simulink model "NetworkModelIntermediateIntersectionRDDSample1"  (R2018b)
settings: Solver=VariableStepAuto  StartTime=0.0  StopTime=10.0  RelTol=1e-3
values from neighbouring files (symbols this model uses):
  Ax = [0 1  0   0 ... (first row only)    [DroneSubsystemModelling.m]
  Ay = [0 1  0   0 ... (first row only)    [DroneSubsystemModelling.m]
  Bx = [0;0;0;b1]    [DroneSubsystemModelling.m]
  By = [0;0;0;b2]    [DroneSubsystemModelling.m]
  ConflictDrone1andDrone2 = ControlDetectionFunction(tout,PositionXDrone1TEST, PositionYDrone1TEST, PositionXDrone2TEST, PositionYDrone2TEST, ConflictDrone1andDrone2)    [ConflictDetectionTEST.m]
  ConflictDrone1andDrone3 = ControlDetectionFunction(tout,PositionXDrone1TEST, PositionYDrone1TEST, PositionXDrone3TEST, PositionYDrone3TEST, ConflictDrone1andDrone3)    [ConflictDetectionTEST.m]
  ConflictDrone1andDrone4 = ControlDetectionFunction(tout,PositionXDrone1TEST, PositionYDrone1TEST, PositionXDrone4TEST, PositionYDrone4TEST, ConflictDrone1andDrone4)    [ConflictDetectionTEST.m]
  ConflictDrone2andDrone3 = ControlDetectionFunction(tout,PositionXDrone2TEST, PositionYDrone2TEST, PositionXDrone3TEST, PositionYDrone3TEST, ConflictDrone2andDrone3)    [ConflictDetectionTEST.m]
  ConflictDrone2andDrone4 = ControlDetectionFunction(tout,PositionXDrone2, PositionYDrone2, PositionXDrone4, PositionYDrone4, ConflictDrone2andDrone4)    [ConflictDetection.m]    (also in ConflictDetectionTEST.m = ControlDetectionFunction(tout,PositionXDrone2TEST, PositionY)
  ConflictDrone3andDrone4 = ControlDetectionFunction(tout,PositionXDrone3TEST, PositionYDrone3TEST, PositionXDrone4TEST, PositionYDrone4TEST, ConflictDrone3andDrone4)    [ConflictDetectionTEST.m]
  Cpx = [1 0 0 0]    [DroneSubsystemModelling.m]
  Cpy = [1 0 0 0]    [DroneSubsystemModelling.m]
  Cvx = [0 1 0 0]    [DroneSubsystemModelling.m]
  Cvy = [0 1 0 0]    [DroneSubsystemModelling.m]
  K1 = 1    [MotionModelling.m]
  K2 = 0.25    [MotionModelling.m]
  K3 = 0.25    [MotionModelling.m]
  K4 = 1    [MotionModelling.m]
  theta1 = -180    [MotionModelling.m]
  theta2 = -3*180/4    (= -135)    [MotionModelling.m]
  theta3 = -2*180/4    (= -90)    [MotionModelling.m]
  theta4 = -180/4    (= -45)    [MotionModelling.m]
  VelocityStarX1 = vx10    [MotionModelling.m]
  VelocityStarX2 = vx20    [MotionModelling.m]
  VelocityStarX3 = vx30    [MotionModelling.m]
  VelocityStarX4 = vx40    [MotionModelling.m]
  VelocityStarY1 = vy10    [MotionModelling.m]
  VelocityStarY2 = vy20    [MotionModelling.m]
  VelocityStarY3 = vy30    [MotionModelling.m]
  VelocityStarY4 = vy40    [MotionModelling.m]
  X10 = [x10 vx10 0 0]'    [MotionModelling.m]
  X20 = [x20 vx20 0 0]'    [MotionModelling.m]
  X30 = [x30 vx30 0 0]'    [MotionModelling.m]
  X40 = [x40 vx40 0 0]'    [MotionModelling.m]
  Y10 = [y10 vy10 0 0]'    [MotionModelling.m]
  Y20 = [y20 vy20 0 0]'    [MotionModelling.m]
  Y30 = [y30 vy30 0 0]'    [MotionModelling.m]
  Y40 = [y40 vy40 0 0]'    [MotionModelling.m]
libraries: simulink x8
settings Model: Creator=CowUser  LastModifiedBy=CowUser

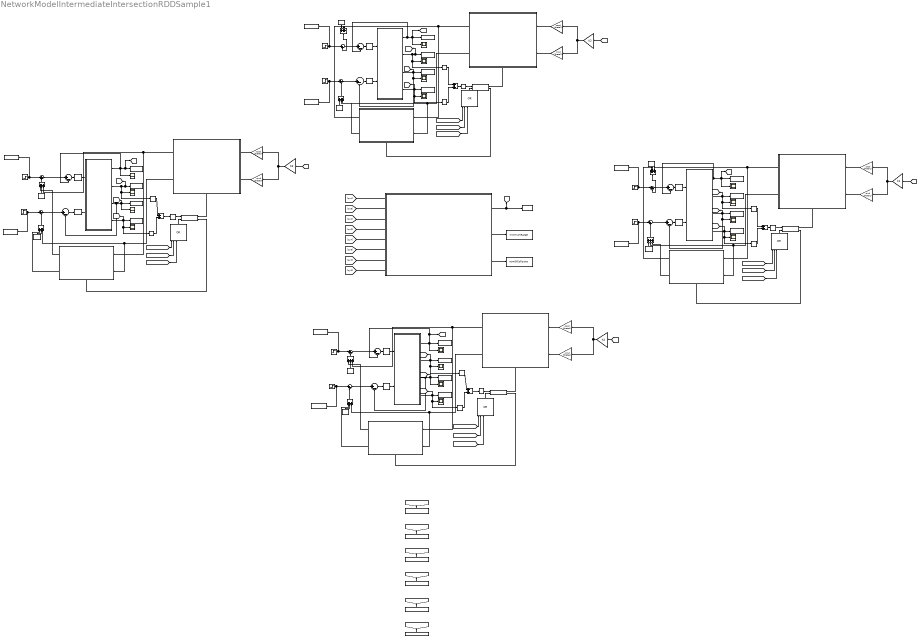
== system NetworkModelIntermediateIntersectionRDDSample1 ==
  note: Drone 3
  note: Drone 1
  note: Drone 2
  note: Drone 4
  note: Sample 4
  note: Sample 2
  note: Sample 1
  note: Sample 3
  note: Sample 5
  note: Sample 6
  Add{7,10..16} (8 alike) : Sum  Inputs=+++
  Add{8..9,17..18} (4 alike) : Sum
  Constant{6..8,10..14} (8 alike) : Constant  Value=0
  Constant25 : Constant  Value=ConflictDrone1andDrone3
  Constant26 : Constant  Value=ConflictDrone1andDrone2
  Constant27 : Constant  Value=ConflictDrone1andDrone4
  Constant28 : Constant  Value=ConflictDrone2andDrone4
  Constant29 : Constant  Value=ConflictDrone3andDrone4
  Constant30 : Constant  Value=ConflictDrone2andDrone3  VectorParams1D=off
  Drone1 Subsystem : Subsystem
  Drone2 Subsystem : Subsystem
  Drone3 Subsystem : Subsystem
  Drone4 Subsystem : Subsystem
  Gain : Gain  Gain=K2
  Gain1 : Gain  Gain=-sind (theta4)
  Gain10 : Gain  Gain=cosd (theta1)
  Gain11 : Gain  Gain=-cosd (theta3)
  Gain12 : Gain  Gain=sind (theta1)
  Gain2 : Gain  Gain=cosd (theta2)
  Gain3 : Gain  Gain=-cosd (theta4)
  Gain4 : Gain  Gain=sind (theta2)
  Gain5 : Gain  Gain=K4
  Gain6 : Gain  Gain=K3
  Gain7 : Gain  Gain=K1
  Gain9 : Gain  Gain=-sind (theta3)
  If Action Subsystem2 : Subsystem  TreatAsAtomicUnit=on
  If Action Subsystem3 : Subsystem  TreatAsAtomicUnit=on
  If Action Subsystem5 : Subsystem  TreatAsAtomicUnit=on
  If Action Subsystem6 : Subsystem  TreatAsAtomicUnit=on
  If{2,4..6} (4 alike) : If  NumInputs=2  IfExpression=(u1 <= R)&(u2 == 1)  ElseIfExpressions=(u1 > R)&(u2 == 1)  ShowElse=off
  MATLAB Function2 : MATLAB Function  TreatAsAtomicUnit=on
  OR{3..6} (4 alike) : Logic  Operator=OR  Inputs=7  IconShape=distinctive  AllPortsSameDT=off  OutDataTypeStr='double'
  PID Controller{2,4..5,8..12} (8 alike) : simulink/Continuous/PID Controller  Controller=PID  Form=Parallel  TimeDomain=Continuous-time  SampleTime=-1  IntegratorMethod=Forward Euler  FilterMethod=Forward Euler  ControllerParametersSource=internal  P=1.97139727738968e-05  I=1.5233344900537e-08  D=0.00566857635684116  UseFilter=on  N=15.1370363747334  TunerSelectOption=Transfer Function Based (PID Tuner App)  InitialConditionSource=internal  InitialConditionForIntegrator=0  InitialConditionForFilter=0  DifferentiatorICPrevScaledInput=0  ExternalReset=none  TrackingMode=off  Kt=1  LimitOutput=off  UpperSaturationLimit=inf  LowerSaturationLimit=-inf  LinearizeAsGain=on  AntiWindupMode=none  Kb=1  POutMin=[]  POutMax=[]  IOutMin=[]  IOutMax=[]  DOutMin=[]  DOutMax=[]  NOutMin=[]  NOutMax=[]  SumOutMin=[]  SumOutMax=[]  SaturationOutMin=[]  SaturationOutMax=[]  PParamMin=[]  PParamMax=[]  IParamMin=[]  IParamMax=[]  DParamMin=[]  DParamMax=[]  NParamMin=[]  NParamMax=[]  KbParamMin=[]  KbParamMax=[]  KtParamMin=[]  KtParamMax=[]  KbOutMin=[]  KbOutMax=[]  KtOutMin=[]  KtOutMax=[]  IntegratorOutMin=[]  IntegratorOutMax=[]  FilterOutMin=[]  FilterOutMax=[]  SumI1OutMin=[]  SumI1OutMax=[]  SumI2OutMin=[]  SumI2OutMax=[]  SumI3OutMin=[]  SumI3OutMax=[]  SumI4OutMin=[]  SumI4OutMax=[]  SumDOutMin=[]  SumDOutMax=[]  DifferentiatorOutMin=[]  DifferentiatorOutMax=[]  FilterDiffOutCoefMin=[]  FilterDiffOutCoefMax=[]  ReciprocalOutMin=[]  ReciprocalOutMax=[]  SumDenOutMin=[]  SumDenOutMax=[]  SumNumOutMin=[]  SumNumOutMax=[]  DivideOutMin=[]  DivideOutMax=[]  IntegratorContinuousStateAttributes=''  IntegratorStateMustResolveToSignalObject=off  IntegratorRTWStateStorageClass=Auto  FilterContinuousStateAttributes=''  FilterStateMustResolveToSignalObject=off  FilterRTWStateStorageClass=Auto  ParallelPVariant=InternalParameters  IdealPVariant=Disabled  IVariant=InternalParameters  DVariant=InternalParameters  IntegratorVariant=Continuous  SatVariant=Disabled  AWVariant=Passthrough  PCopyVariant=Disabled  TRVariant=Disabled  FdbkBlocksVariant=Forward  IdealPFdbkVariant=Disabled  SatFdbkVariant=Disabled  DerivativeFilterVariant=ContFilter  NVariant=InternalParameters  NCopyVariant=Disabled  FilterICVariant=InternalICsFilter  IntegratorICVariant=InternalICs  ExternalResetVariant=Disabled  TRSumVariant=Passthrough  SumFdbkVariant=Disabled  SumVariant=Sum_PID
  PositionXDrone{1..4} (4 alike) : Scope
  PositionYDrone{1..4} (4 alike) : Scope
  Sqrt{3..6} (4 alike) : Sqrt  SaturateOnIntegerOverflow=on
  Square{5..12} (8 alike) : Math  Operator=square  SaturateOnIntegerOverflow=on
  Step 10 : Step  Time=0  After=VelocityStarY1  SampleTime=0
  Step 11 : Step  Time=0  After=VelocityStarX3  SampleTime=0
  Step 12 : Step  Time=0  After=VelocityStarY3  SampleTime=0
  Step 3 : Step  Time=0  After=VelocityStarX2  SampleTime=0
  Step 4 : Step  Time=0  After=VelocityStarY2  SampleTime=0
  Step 5 : Step  Time=0  After=VelocityStarX4  SampleTime=0
  Step 6 : Step  Time=0  After=VelocityStarY4  SampleTime=0
  Step 9 : Step  Time=0  After=VelocityStarX1  SampleTime=0
  Sum{9..24} (16 alike) : Sum  Inputs=|+-
  Switch Case Action Subsystem : Subsystem  TreatAsAtomicUnit=on
  Switch Case Action Subsystem1 : Subsystem  TreatAsAtomicUnit=on
  Switch Case Action Subsystem4 : Subsystem  TreatAsAtomicUnit=on
  Switch Case Action Subsystem5 : Subsystem  TreatAsAtomicUnit=on
  To Workspace10 : ToWorkspace  VariableName=VelocityYDrone4  SampleTime=-1
  To Workspace11 : ToWorkspace  VariableName=PositionXDrone4  SampleTime=-1
  To Workspace12 : ToWorkspace  VariableName=VelocityXDrone4  SampleTime=-1
  To Workspace13 : ToWorkspace  VariableName=VelocityStarX4  SampleTime=-1
  To Workspace14 : ToWorkspace  VariableName=PositionYDrone4  SampleTime=-1
  To Workspace15 : ToWorkspace  VariableName=PositionXDrone2  SampleTime=-1
  To Workspace16 : ToWorkspace  VariableName=VelocityXDrone2  SampleTime=-1
  To Workspace17 : ToWorkspace  VariableName=VelocityStarX2  SampleTime=-1
  To Workspace18 : ToWorkspace  VariableName=PositionYDrone2  SampleTime=-1
  To Workspace25 : ToWorkspace  VariableName=VelocityYDrone3  SampleTime=-1
  To Workspace26 : ToWorkspace  VariableName=VelocityXDrone1  SampleTime=-1
  To Workspace27 : ToWorkspace  VariableName=PositionXDrone3  SampleTime=-1
  To Workspace28 : ToWorkspace  VariableName=VelocityStarX1  SampleTime=-1
  To Workspace29 : ToWorkspace  VariableName=PositionYDrone1  SampleTime=-1
  To Workspace30 : ToWorkspace  VariableName=VelocityStarY1  SampleTime=-1
  To Workspace31 : ToWorkspace  VariableName=VelocityStarY3  SampleTime=-1
  To Workspace32 : ToWorkspace  VariableName=VelocityYDrone1  SampleTime=-1
  To Workspace33 : ToWorkspace  VariableName=VelocityXDrone3  SampleTime=-1
  To Workspace34 : ToWorkspace  VariableName=VelocityStarX3  SampleTime=-1
  To Workspace35 : ToWorkspace  VariableName=PositionYDrone3  SampleTime=-1
  To Workspace36 : ToWorkspace  VariableName=PositionXDrone1  SampleTime=-1
  To Workspace49 : ToWorkspace  VariableName=Vdiff  SampleTime=-1
  To Workspace53 : ToWorkspace  VariableName=minimumRange  SampleTime=-1
  To Workspace54 : ToWorkspace  VariableName=numOfCollisions  SampleTime=-1
  To Workspace7 : ToWorkspace  VariableName=VelocityStarY2  SampleTime=-1
  To Workspace8 : ToWorkspace  VariableName=VelocityStarY4  SampleTime=-1
  To Workspace9 : ToWorkspace  VariableName=VelocityYDrone2  SampleTime=-1
  VelocityXDrone{1..4} (4 alike) : Scope
  VelocityYDrone{1..4} (4 alike) : Scope
  wires:
  Drone3 Subsystem/3(Vy) -> Sum21/2, [qDotyC], VelocityYDrone3/1, To Workspace25/1
  Sum16/1 -> PID Controller5/1
  If6/1 -> If Action Subsystem5/Action
  Gain10/1 -> If Action Subsystem5/1(deltaVx1)
  Sum22/1 -> Sum12/1
  Constant11/1 -> Add10/1
  Constant7/1 -> Add7/1
  Square8/1 -> Add8/1
  Drone4 Subsystem/3(Vy) -> Sum17/2, [qDotyD], VelocityYDrone4/1, To Workspace10/1
  PID Controller10/1 -> Drone3 Subsystem/2("InputForceY* ")
  If Action Subsystem3/2(dVy4) -> Switch Case Action Subsystem1/2(deltaVy4), Add13/3
  Drone2 Subsystem/2(x) -> [qxB], To Workspace15/1, Square8/1, PositionXDrone2/1
  PID Controller2/1 -> Drone2 Subsystem/2("InputForceY* ")
  [qxC] -> MATLAB Function2/3(qxC)
  Step 5/1 -> Sum18/1, To Workspace13/1
  Add13/1 -> Sum19/2
  Add14/1 -> Sum24/2
  Step 11/1 -> Sum22/1, To Workspace34/1
  Sqrt4/1 -> If4/1
  Switch Case Action Subsystem4/2(dVy1) -> Add7/3
  If4/2 -> Switch Case Action Subsystem/Action
  PID Controller4/1 -> Drone4 Subsystem/2("InputForceY* ")
  Add11/1 -> Sum20/2
  Add17/1 -> Sqrt3/1
  Gain3/1 -> If Action Subsystem3/1(deltaVx4)
  Constant8/1 -> Add15/2
  Square5/1 -> Add18/1
  Sum21/1 -> PID Controller10/1
  Switch Case Action Subsystem5/2(dVy3) -> Add16/1
  Sqrt3/1 -> If6/1
  Step 4/1 -> Sum14/1, To Workspace7/1
  Gain12/1 -> If Action Subsystem5/2(deltaVy1)
  Step 12/1 -> To Workspace31/1, Sum23/1
  Switch Case Action Subsystem4/1(dVx1) -> Add14/1
  OR5/1 -> If5/2
  Sum11/1 -> PID Controller12/1
  If5/2 -> Switch Case Action Subsystem5/Action
  Drone3 Subsystem/2(x) -> Square5/1, PositionXDrone3/1, [qxC], To Workspace27/1
  Drone1 Subsystem/2(x) -> [qxA], Square7/1, PositionXDrone1/1, To Workspace36/1
  MATLAB Function2/2(minimumRange) -> To Workspace53/1
  Constant6/1 -> Add14/2
  Switch Case Action Subsystem/2(dVy2) -> Add10/3
  Step 10/1 -> Sum10/1, To Workspace30/1
  Add15/1 -> Sum22/2
  Sum24/1 -> Sum11/1
  If5/1 -> If Action Subsystem6/Action
  Drone4 Subsystem/4(y) -> [qyD], Square11/1, PositionYDrone4/1, To Workspace14/1
  Sum10/1 -> Sum9/1
  Constant14/1 -> Add16/2
  PID Controller12/1 -> Drone1 Subsystem/1(InputForceX*)
  Drone1 Subsystem/1(Vx) -> [qDotxA], VelocityXDrone1/1, To Workspace26/1, Sum11/2
  OR4/1 -> If4/2
  Drone4 Subsystem/2(x) -> Square10/1, PositionXDrone4/1, To Workspace11/1, [qxD]
  Sqrt5/1 -> If2/1
  Switch Case Action Subsystem1/1(dVx4) -> Add12/1
  If6/2 -> Switch Case Action Subsystem4/Action
  Drone2 Subsystem/3(Vy) -> [qDotyB], To Workspace9/1, Sum13/2, VelocityYDrone2/1
  [qxB] -> MATLAB Function2/2(qxB)
  If Action Subsystem6/2(dVy3) -> Switch Case Action Subsystem5/2(deltaVy3), Add16/3
  If4/1 -> If Action Subsystem2/Action
  [qyA] -> MATLAB Function2/5(qyA)
  Add16/1 -> Sum23/2
  [qyB] -> MATLAB Function2/6(qyB)
  [qxD] -> MATLAB Function2/4(qxD)
  Add10/1 -> Sum14/2
  Add7/1 -> Sum10/2
  Sum18/1 -> Sum16/1
  Drone1 Subsystem/3(Vy) -> [qDotyA], To Workspace32/1, Sum9/2, VelocityYDrone1/1
  PID Controller9/1 -> Drone1 Subsystem/2("InputForceY* ")
  If Action Subsystem5/2(dVy1) -> Add7/2, Switch Case Action Subsystem4/2(deltaVy1)
  Gain9/1 -> If Action Subsystem6/2(deltaVy3)
  Gain11/1 -> If Action Subsystem6/1(deltaVx3)
  Sum9/1 -> PID Controller9/1
  Square11/1 -> Add9/2
  Sqrt6/1 -> If5/1
  Sum15/1 -> PID Controller8/1
  OR6/1 -> If6/2
  Drone1 Subsystem/4(y) -> [qyA], To Workspace29/1, Square12/1, PositionYDrone1/1
  PID Controller8/1 -> Drone2 Subsystem/1(InputForceX*)
  Add8/1 -> Sqrt4/1
  Gain4/1 -> If Action Subsystem2/2(deltaVy2)
  If Action Subsystem5/1(dVx1) -> Switch Case Action Subsystem4/1(deltaVx1), Add14/3
  Gain2/1 -> If Action Subsystem2/1(deltaVx2)
  Sum19/1 -> Sum17/1
  Sum14/1 -> Sum13/1
  Gain1/1 -> If Action Subsystem3/2(deltaVy4)
  If Action Subsystem2/2(dVy2) -> Add10/2, Switch Case Action Subsystem/2(deltaVy2)
  If2/2 -> Switch Case Action Subsystem1/Action
  Sum17/1 -> PID Controller4/1
  Add18/1 -> Sqrt6/1
  Sum20/1 -> Sum15/1
  Step 3/1 -> Sum20/1, To Workspace17/1
  Drone3 Subsystem/4(y) -> [qyC], Square6/1, PositionYDrone3/1, To Workspace35/1
  [ConflictDrone2andDrone4] -> OR4/3
  [ConflictDrone2andDrone3] -> OR4/2
  [qxA] -> MATLAB Function2/1(qxA)
  Square6/1 -> Add18/2
  If Action Subsystem6/1(dVx3) -> Switch Case Action Subsystem5/1(deltaVx3), Add15/3
  Sum12/1 -> PID Controller11/1
  If Action Subsystem3/1(dVx4) -> Switch Case Action Subsystem1/1(deltaVx4), Add12/3
  Add12/1 -> Sum18/2
  Constant10/1 -> Add11/2
  If Action Subsystem2/1(dVx2) -> Switch Case Action Subsystem/1(deltaVx2), Add11/3
  [ConflictDrone1andDrone2] -> OR4/1
  OR3/1 -> If2/2
  PID Controller5/1 -> Drone4 Subsystem/1(InputForceX*)
  Drone2 Subsystem/4(y) -> [qyB], To Workspace18/1, Square9/1, PositionYDrone2/1
  Drone2 Subsystem/1(Vx) -> Sum15/2, [qDotxB], VelocityXDrone2/1, To Workspace16/1
  Step 9/1 -> Sum24/1, To Workspace28/1
  Square9/1 -> Add8/2
  [qyD] -> MATLAB Function2/8(qyD)
  Switch Case Action Subsystem5/1(dVx3) -> Add15/1
  [qyC] -> MATLAB Function2/7(qyC)
  Switch Case Action Subsystem/1(dVx2) -> Add11/1
  [ConflictDrone1andDrone2] -> OR6/2
  If2/1 -> If Action Subsystem3/Action
  Drone4 Subsystem/1(Vx) -> [qDotxD], Sum16/2, To Workspace12/1, VelocityXDrone4/1
  Sum13/1 -> PID Controller2/1
  PID Controller11/1 -> Drone3 Subsystem/1(InputForceX*)
  [ConflictDrone2andDrone3] -> OR5/2
  Drone3 Subsystem/1(Vx) -> Sum12/2, [qDotxC], To Workspace33/1, VelocityXDrone3/1
  Constant13/1 -> Add13/2
  Constant12/1 -> Add12/2
  Switch Case Action Subsystem1/2(dVy4) -> Add13/1
  Square12/1 -> Add17/2
  Add9/1 -> Sqrt5/1
  Step 6/1 -> To Workspace8/1, Sum19/1
  Square10/1 -> Add9/1
  Sum23/1 -> Sum21/1
  Square7/1 -> Add17/1
  [ConflictDrone1andDrone4] -> OR6/3
  [ConflictDrone1andDrone3] -> OR6/1
  [ConflictDrone3andDrone4] -> OR5/3
  [ConflictDrone1andDrone3] -> OR5/1
  [ConflictDrone1andDrone4] -> OR3/1
  [ConflictDrone2andDrone4] -> OR3/2
  MATLAB Function2/3(numOfCollisions) -> To Workspace54/1
  Constant28/1 -> [ConflictDrone2andDrone4]
  Constant26/1 -> [ConflictDrone1andDrone2]
  Constant30/1 -> [ConflictDrone2andDrone3]
  Constant27/1 -> [ConflictDrone1andDrone4]
  Constant29/1 -> [ConflictDrone3andDrone4]
  Constant25/1 -> [ConflictDrone1andDrone3]
  Gain/1 -> Gain4/1, Gain2/1
  Gain5/1 -> Gain1/1, Gain3/1
  Gain6/1 -> Gain9/1, Gain11/1
  Gain7/1 -> Gain10/1, Gain12/1
  [Vdiff] -> Gain/1
  [Vdiff] -> Gain5/1
  [Vdiff] -> Gain6/1
  [Vdiff] -> Gain7/1
  MATLAB Function2/1(Vdiff) -> [Vdiff], To Workspace49/1
  [ConflictDrone3andDrone4] -> OR3/3

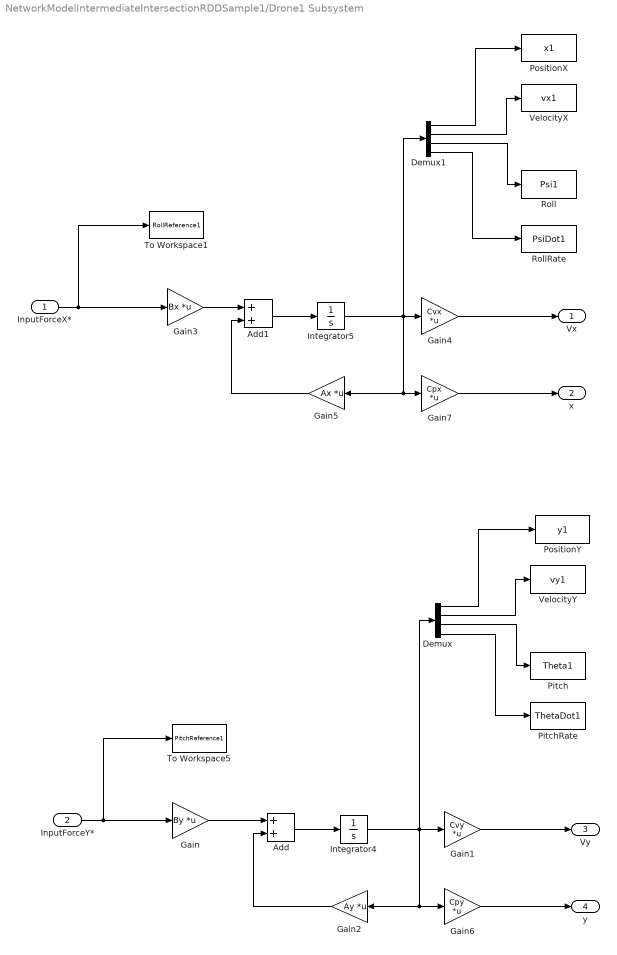
== system NetworkModelIntermediateIntersectionRDDSample1/Drone1 Subsystem ==
  InputForceX* : Inport
  "InputForceY* " : Inport  Port=2
  Add : Sum
  Add1 : Sum
  Demux : Demux
  Demux1 : Demux
  Gain : Gain  Gain=By  Multiplication=Matrix(K*u)
  Gain1 : Gain  Gain=Cvy  Multiplication=Matrix(K*u)
  Gain2 : Gain  Gain=Ay  Multiplication=Matrix(K*u)
  Gain3 : Gain  Gain=Bx  Multiplication=Matrix(K*u)
  Gain4 : Gain  Gain=Cvx  Multiplication=Matrix(K*u)
  Gain5 : Gain  Gain=Ax  Multiplication=Matrix(K*u)
  Gain6 : Gain  Gain=Cpy  Multiplication=Matrix(K*u)
  Gain7 : Gain  Gain=Cpx  Multiplication=Matrix(K*u)
  Integrator4 : Integrator  InitialCondition=Y10
  Integrator5 : Integrator  InitialCondition=X10
  Pitch : ToWorkspace  VariableName=Theta1  SampleTime=-1
  PitchRate : ToWorkspace  VariableName=ThetaDot1  SampleTime=-1
  PositionX : ToWorkspace  VariableName=x1  SampleTime=-1
  PositionY : ToWorkspace  VariableName=y1  SampleTime=-1
  Roll : ToWorkspace  VariableName=Psi1  SampleTime=-1
  RollRate : ToWorkspace  VariableName=PsiDot1  SampleTime=-1
  To Workspace1 : ToWorkspace  VariableName=RollReference1  SampleTime=-1
  To Workspace5 : ToWorkspace  VariableName=PitchReference1  SampleTime=-1
  VelocityX : ToWorkspace  VariableName=vx1  SampleTime=-1
  VelocityY : ToWorkspace  VariableName=vy1  SampleTime=-1
  Vx : Outport
  x : Outport  Port=2
  Vy : Outport  Port=3
  y : Outport  Port=4
  wires:
  Demux/1 -> PositionY/1
  Demux1/2 -> VelocityX/1
  Demux1/4 -> RollRate/1
  Demux1/3 -> Roll/1
  Gain4/1 -> Vx/1
  "InputForceY* "/1 -> Gain/1, To Workspace5/1
  Gain/1 -> Add/1
  Demux/4 -> PitchRate/1
  Demux/3 -> Pitch/1
  Add/1 -> Integrator4/1
  Demux1/1 -> PositionX/1
  Gain1/1 -> Vy/1
  InputForceX*/1 -> Gain3/1, To Workspace1/1
  Gain7/1 -> x/1
  Integrator4/1 -> Gain6/1, Gain2/1, Demux/1, Gain1/1
  Demux/2 -> VelocityY/1
  Gain6/1 -> y/1
  Gain3/1 -> Add1/1
  Add1/1 -> Integrator5/1
  Gain2/1 -> Add/2
  Integrator5/1 -> Gain4/1, Gain5/1, Gain7/1, Demux1/1
  Gain5/1 -> Add1/2

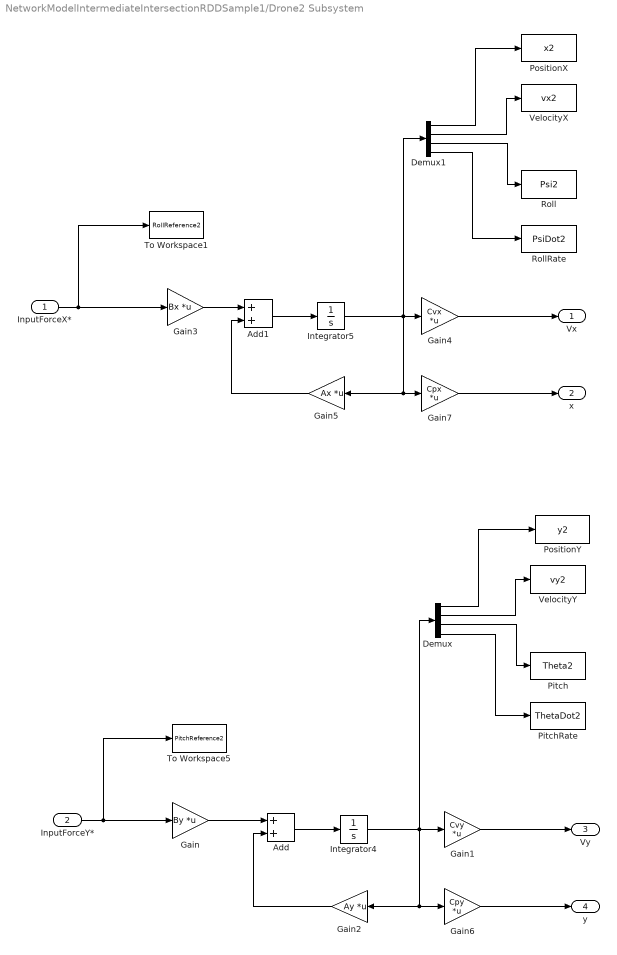
== system NetworkModelIntermediateIntersectionRDDSample1/Drone2 Subsystem ==
  InputForceX* : Inport
  "InputForceY* " : Inport  Port=2
  Add : Sum
  Add1 : Sum
  Demux : Demux
  Demux1 : Demux
  Gain : Gain  Gain=By  Multiplication=Matrix(K*u)
  Gain1 : Gain  Gain=Cvy  Multiplication=Matrix(K*u)
  Gain2 : Gain  Gain=Ay  Multiplication=Matrix(K*u)
  Gain3 : Gain  Gain=Bx  Multiplication=Matrix(K*u)
  Gain4 : Gain  Gain=Cvx  Multiplication=Matrix(K*u)
  Gain5 : Gain  Gain=Ax  Multiplication=Matrix(K*u)
  Gain6 : Gain  Gain=Cpy  Multiplication=Matrix(K*u)
  Gain7 : Gain  Gain=Cpx  Multiplication=Matrix(K*u)
  Integrator4 : Integrator  InitialCondition=Y20
  Integrator5 : Integrator  InitialCondition=X20
  Pitch : ToWorkspace  VariableName=Theta2  SampleTime=-1
  PitchRate : ToWorkspace  VariableName=ThetaDot2  SampleTime=-1
  PositionX : ToWorkspace  VariableName=x2  SampleTime=-1
  PositionY : ToWorkspace  VariableName=y2  SampleTime=-1
  Roll : ToWorkspace  VariableName=Psi2  SampleTime=-1
  RollRate : ToWorkspace  VariableName=PsiDot2  SampleTime=-1
  To Workspace1 : ToWorkspace  VariableName=RollReference2  SampleTime=-1
  To Workspace5 : ToWorkspace  VariableName=PitchReference2  SampleTime=-1
  VelocityX : ToWorkspace  VariableName=vx2  SampleTime=-1
  VelocityY : ToWorkspace  VariableName=vy2  SampleTime=-1
  Vx : Outport
  x : Outport  Port=2
  Vy : Outport  Port=3
  y : Outport  Port=4
  wires:
  Demux/1 -> PositionY/1
  Demux1/2 -> VelocityX/1
  Demux1/4 -> RollRate/1
  Demux1/3 -> Roll/1
  Gain4/1 -> Vx/1
  "InputForceY* "/1 -> Gain/1, To Workspace5/1
  Gain/1 -> Add/1
  Demux/4 -> PitchRate/1
  Demux/3 -> Pitch/1
  Add/1 -> Integrator4/1
  Demux1/1 -> PositionX/1
  Gain1/1 -> Vy/1
  InputForceX*/1 -> Gain3/1, To Workspace1/1
  Gain7/1 -> x/1
  Integrator4/1 -> Gain6/1, Gain2/1, Demux/1, Gain1/1
  Demux/2 -> VelocityY/1
  Gain6/1 -> y/1
  Gain3/1 -> Add1/1
  Add1/1 -> Integrator5/1
  Gain2/1 -> Add/2
  Integrator5/1 -> Gain4/1, Gain5/1, Gain7/1, Demux1/1
  Gain5/1 -> Add1/2

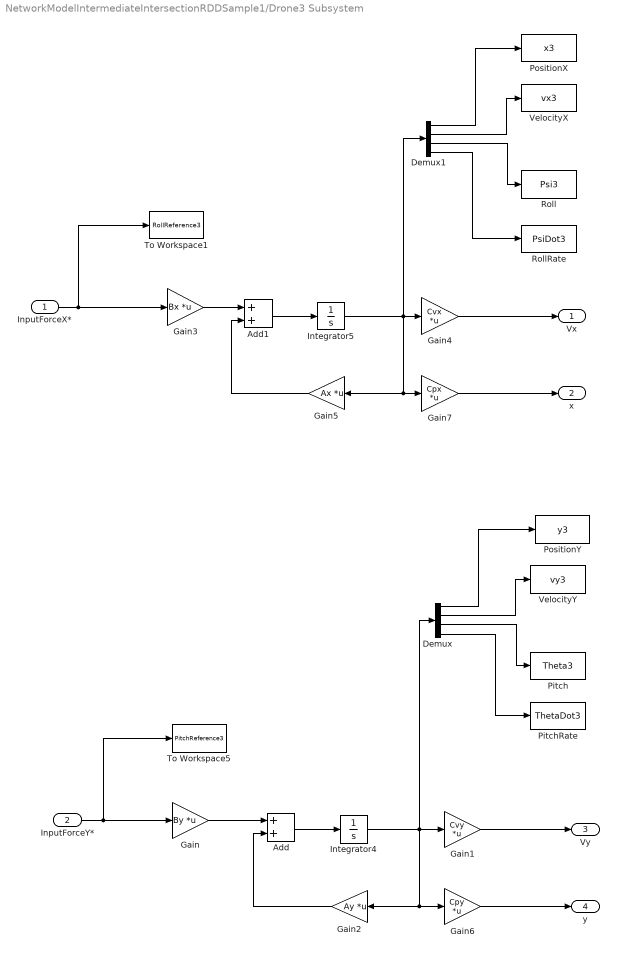
== system NetworkModelIntermediateIntersectionRDDSample1/Drone3 Subsystem ==
  InputForceX* : Inport
  "InputForceY* " : Inport  Port=2
  Add : Sum
  Add1 : Sum
  Demux : Demux
  Demux1 : Demux
  Gain : Gain  Gain=By  Multiplication=Matrix(K*u)
  Gain1 : Gain  Gain=Cvy  Multiplication=Matrix(K*u)
  Gain2 : Gain  Gain=Ay  Multiplication=Matrix(K*u)
  Gain3 : Gain  Gain=Bx  Multiplication=Matrix(K*u)
  Gain4 : Gain  Gain=Cvx  Multiplication=Matrix(K*u)
  Gain5 : Gain  Gain=Ax  Multiplication=Matrix(K*u)
  Gain6 : Gain  Gain=Cpy  Multiplication=Matrix(K*u)
  Gain7 : Gain  Gain=Cpx  Multiplication=Matrix(K*u)
  Integrator4 : Integrator  InitialCondition=Y30
  Integrator5 : Integrator  InitialCondition=X30
  Pitch : ToWorkspace  VariableName=Theta3  SampleTime=-1
  PitchRate : ToWorkspace  VariableName=ThetaDot3  SampleTime=-1
  PositionX : ToWorkspace  VariableName=x3  SampleTime=-1
  PositionY : ToWorkspace  VariableName=y3  SampleTime=-1
  Roll : ToWorkspace  VariableName=Psi3  SampleTime=-1
  RollRate : ToWorkspace  VariableName=PsiDot3  SampleTime=-1
  To Workspace1 : ToWorkspace  VariableName=RollReference3  SampleTime=-1
  To Workspace5 : ToWorkspace  VariableName=PitchReference3  SampleTime=-1
  VelocityX : ToWorkspace  VariableName=vx3  SampleTime=-1
  VelocityY : ToWorkspace  VariableName=vy3  SampleTime=-1
  Vx : Outport
  x : Outport  Port=2
  Vy : Outport  Port=3
  y : Outport  Port=4
  wires:
  Gain4/1 -> Vx/1
  Demux/2 -> VelocityY/1
  Demux/4 -> PitchRate/1
  Gain3/1 -> Add1/1
  InputForceX*/1 -> Gain3/1, To Workspace1/1
  Gain2/1 -> Add/2
  Demux1/3 -> Roll/1
  Gain7/1 -> x/1
  Add1/1 -> Integrator5/1
  Demux/3 -> Pitch/1
  Gain5/1 -> Add1/2
  Gain6/1 -> y/1
  Integrator5/1 -> Gain4/1, Gain5/1, Gain7/1, Demux1/1
  Gain/1 -> Add/1
  Demux/1 -> PositionY/1
  Add/1 -> Integrator4/1
  Demux1/4 -> RollRate/1
  "InputForceY* "/1 -> Gain/1, To Workspace5/1
  Integrator4/1 -> Gain6/1, Gain2/1, Demux/1, Gain1/1
  Demux1/1 -> PositionX/1
  Demux1/2 -> VelocityX/1
  Gain1/1 -> Vy/1

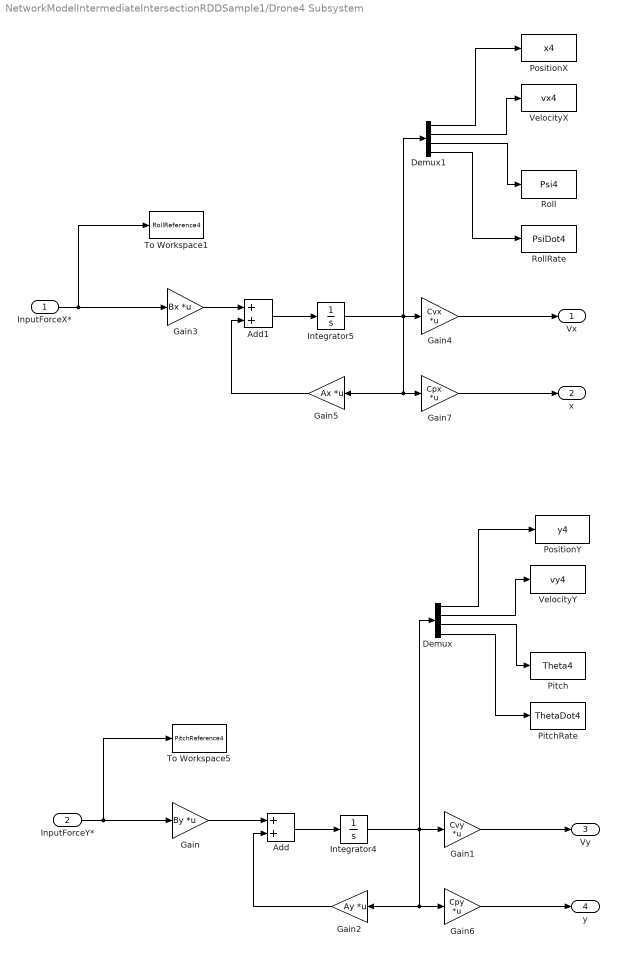
== system NetworkModelIntermediateIntersectionRDDSample1/Drone4 Subsystem ==
  InputForceX* : Inport
  "InputForceY* " : Inport  Port=2
  Add : Sum
  Add1 : Sum
  Demux : Demux
  Demux1 : Demux
  Gain : Gain  Gain=By  Multiplication=Matrix(K*u)
  Gain1 : Gain  Gain=Cvy  Multiplication=Matrix(K*u)
  Gain2 : Gain  Gain=Ay  Multiplication=Matrix(K*u)
  Gain3 : Gain  Gain=Bx  Multiplication=Matrix(K*u)
  Gain4 : Gain  Gain=Cvx  Multiplication=Matrix(K*u)
  Gain5 : Gain  Gain=Ax  Multiplication=Matrix(K*u)
  Gain6 : Gain  Gain=Cpy  Multiplication=Matrix(K*u)
  Gain7 : Gain  Gain=Cpx  Multiplication=Matrix(K*u)
  Integrator4 : Integrator  InitialCondition=Y40
  Integrator5 : Integrator  InitialCondition=X40
  Pitch : ToWorkspace  VariableName=Theta4  SampleTime=-1
  PitchRate : ToWorkspace  VariableName=ThetaDot4  SampleTime=-1
  PositionX : ToWorkspace  VariableName=x4  SampleTime=-1
  PositionY : ToWorkspace  VariableName=y4  SampleTime=-1
  Roll : ToWorkspace  VariableName=Psi4  SampleTime=-1
  RollRate : ToWorkspace  VariableName=PsiDot4  SampleTime=-1
  To Workspace1 : ToWorkspace  VariableName=RollReference4  SampleTime=-1
  To Workspace5 : ToWorkspace  VariableName=PitchReference4  SampleTime=-1
  VelocityX : ToWorkspace  VariableName=vx4  SampleTime=-1
  VelocityY : ToWorkspace  VariableName=vy4  SampleTime=-1
  Vx : Outport
  x : Outport  Port=2
  Vy : Outport  Port=3
  y : Outport  Port=4
  wires:
  Gain4/1 -> Vx/1
  Demux/2 -> VelocityY/1
  Demux/4 -> PitchRate/1
  Gain3/1 -> Add1/1
  InputForceX*/1 -> Gain3/1, To Workspace1/1
  Gain2/1 -> Add/2
  Demux1/3 -> Roll/1
  Gain7/1 -> x/1
  Add1/1 -> Integrator5/1
  Demux/3 -> Pitch/1
  Gain5/1 -> Add1/2
  Gain6/1 -> y/1
  Integrator5/1 -> Gain4/1, Gain5/1, Gain7/1, Demux1/1
  Gain/1 -> Add/1
  Demux/1 -> PositionY/1
  Add/1 -> Integrator4/1
  Demux1/4 -> RollRate/1
  "InputForceY* "/1 -> Gain/1, To Workspace5/1
  Integrator4/1 -> Gain6/1, Gain2/1, Demux/1, Gain1/1
  Demux1/1 -> PositionX/1
  Demux1/2 -> VelocityX/1
  Gain1/1 -> Vy/1

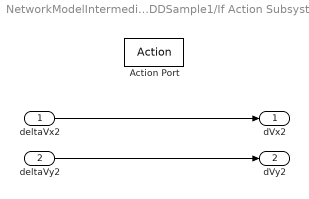
== system NetworkModelIntermediateIntersectionRDDSample1/If Action Subsystem2 ==
  deltaVx2 : Inport
  deltaVy2 : Inport  Port=2
  Action Port : ActionPort  ActionType=then
  dVx2 : Outport
  dVy2 : Outport  Port=2
  wires:
  deltaVx2/1 -> dVx2/1
  deltaVy2/1 -> dVy2/1

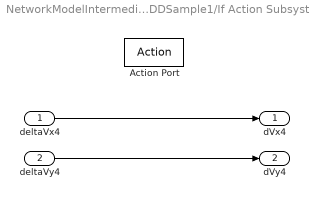
== system NetworkModelIntermediateIntersectionRDDSample1/If Action Subsystem3 ==
  deltaVx4 : Inport
  deltaVy4 : Inport  Port=2
  Action Port : ActionPort  ActionType=then
  dVx4 : Outport
  dVy4 : Outport  Port=2
  wires:
  deltaVx4/1 -> dVx4/1
  deltaVy4/1 -> dVy4/1

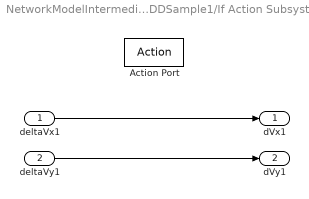
== system NetworkModelIntermediateIntersectionRDDSample1/If Action Subsystem5 ==
  deltaVx1 : Inport
  deltaVy1 : Inport  Port=2
  Action Port : ActionPort  ActionType=then
  dVx1 : Outport
  dVy1 : Outport  Port=2
  wires:
  deltaVx1/1 -> dVx1/1
  deltaVy1/1 -> dVy1/1

== system NetworkModelIntermediateIntersectionRDDSample1/If Action Subsystem6 ==
  deltaVx3 : Inport
  deltaVy3 : Inport  Port=2
  Action Port : ActionPort  ActionType=then
  dVx3 : Outport
  dVy3 : Outport  Port=2
  wires:
  deltaVx3/1 -> dVx3/1
  deltaVy3/1 -> dVy3/1

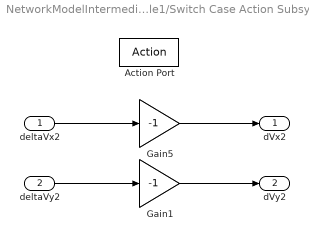
== system NetworkModelIntermediateIntersectionRDDSample1/Switch Case Action Subsystem ==
  deltaVx2 : Inport
  deltaVy2 : Inport  Port=2
  Action Port : ActionPort  ActionType=elseif
  Gain1 : Gain  Gain=-1
  Gain5 : Gain  Gain=-1
  dVx2 : Outport
  dVy2 : Outport  Port=2
  wires:
  deltaVy2/1 -> Gain1/1
  deltaVx2/1 -> Gain5/1
  Gain5/1 -> dVx2/1
  Gain1/1 -> dVy2/1

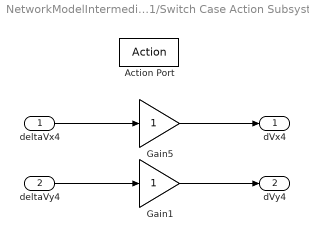
== system NetworkModelIntermediateIntersectionRDDSample1/Switch Case Action Subsystem1 ==
  deltaVx4 : Inport
  deltaVy4 : Inport  Port=2
  Action Port : ActionPort  ActionType=elseif
  Gain1 : Gain
  Gain5 : Gain
  dVx4 : Outport
  dVy4 : Outport  Port=2
  wires:
  deltaVy4/1 -> Gain1/1
  deltaVx4/1 -> Gain5/1
  Gain5/1 -> dVx4/1
  Gain1/1 -> dVy4/1

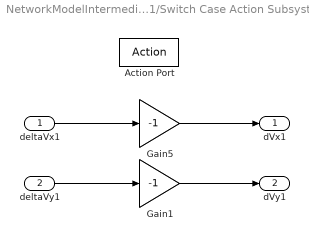
== system NetworkModelIntermediateIntersectionRDDSample1/Switch Case Action Subsystem4 ==
  deltaVx1 : Inport
  deltaVy1 : Inport  Port=2
  Action Port : ActionPort  ActionType=elseif
  Gain1 : Gain  Gain=-1
  Gain5 : Gain  Gain=-1
  dVx1 : Outport
  dVy1 : Outport  Port=2
  wires:
  deltaVy1/1 -> Gain1/1
  deltaVx1/1 -> Gain5/1
  Gain5/1 -> dVx1/1
  Gain1/1 -> dVy1/1

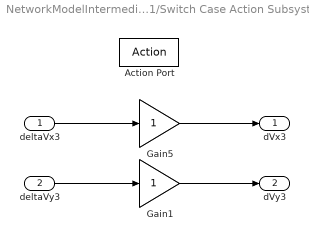
== system NetworkModelIntermediateIntersectionRDDSample1/Switch Case Action Subsystem5 ==
  deltaVx3 : Inport
  deltaVy3 : Inport  Port=2
  Action Port : ActionPort  ActionType=elseif
  Gain1 : Gain
  Gain5 : Gain
  dVx3 : Outport
  dVy3 : Outport  Port=2
  wires:
  deltaVy3/1 -> Gain1/1
  deltaVx3/1 -> Gain5/1
  Gain5/1 -> dVx3/1
  Gain1/1 -> dVy3/1

== matlab function NetworkModelIntermediateIntersectionRDDSample1/MATLAB Function2 ==
  data: qxA input; Vdiff output; qxB input; qxC input; qxD input; qyA input; qyB input; qyC input; qyD input; minimumRange output; numOfCollisions output
function [Vdiff, minimumRange, numOfCollisions] = SpeedController(qxA,qxB,qxC,qxD, qyA, qyB, qyC, qyD)


qx = [qxA, qxB,qxC,qxD];
qy = [qyA, qyB, qyC, qyD];

Vmax = 0.2;

K = 0.25; 
nT = length(qx);
RangeVector = zeros(1,6);
R = 5;

  for k = 1:nT
      
      if sqrt(qx(k)^2 + qy(k)^2) <=  R

        collisionNumber = 0;

            for m = 1:nT

               for n = 1:nT

                   if n > m

                        qxi = qx(m);
                        qyi = qy(m);
                        qxj = qx(n);
                        qyj = qy(n);

                        Range = K*sqrt((qxi - qxj)^2 + (qyi - qyj)^2); 
                      
                        collisionNumber = collisionNumber + 1;
                        
                        RangeVector(collisionNumber) = Range;

                   end 

               end 

            end
           
           minimumRange = min(RangeVector);

           Vdiff = K/minimumRange;
            
           numOfCollisions = collisionNumber;
      else
          
            Vdiff = 0;
            minimumRange = 0;
            numOfCollisions = 0;
      end 
  end 

%     if abs(Vdiff) >= Vmax/2
%         Vdiff = Vmax/2;
%     end 

end
